simulink model "couple"  (R2024b)
settings: Solver=VariableStepAuto  StartTime=0.0  StopTime=10.0  RelTol=1e-3
undefined symbols (not defined in the file): rational, S, sparameters
libraries: simrfV2util1 x3, simrfV2elements x1, simrfV2junction1 x1, simrfV2sources1 x1

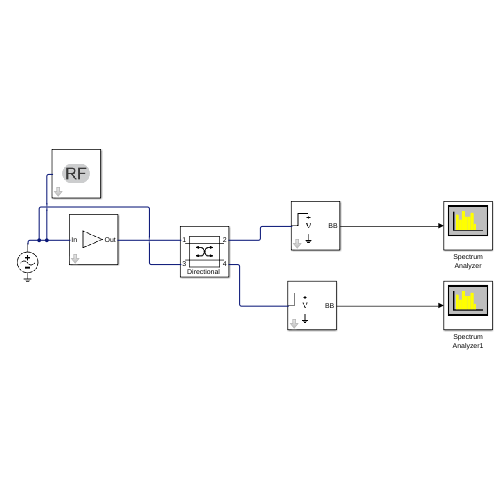
[thumbnail: Simulink's stored preview of the top-level diagram]
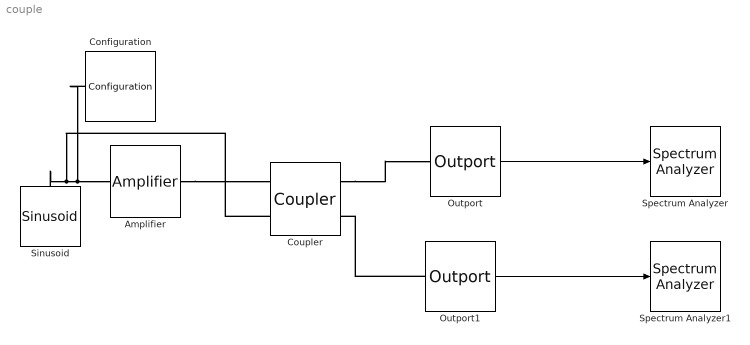
== system couple ==
  Amplifier : simrfV2elements/Amplifier  classname=amplifier  DataSource=Data file  File=unitygain.s2p  isNetworkObj=off  NetworkObject=sparameters('default.s2p')  Paramtype=S-parameters  Sparam=[0 0;1 0]  SparamFreq=1e9 Hz  SparamZ0=50  isRationalObj=off  RationalObject=rational('default.s2p')  Residues=0  Poles=0  DF={0 0; 1 0}  Source_linear_gain=Available power gain  linear_gain=100 dB  AmAmAmPmTable=[-25,5,-1;-10,20,-2;0,27,5;5,28,12]  Zin=50  Zout=50  Source_Poly=Even and odd order  Poly_Coeffs=[0 1]  IPType=Output  IP2=inf dBm  IP3=inf dBm  P1dB=inf dBm  Psat=inf dBm  Gcomp=inf dBm  InternalGrounding=on  SourceFreq=Extracted from data source  PlotFreq=[1e9:1e6:3e9] Hz  PlotType=X-Y plane  YParam1=S(1,1)  YFormat1=Magnitude (dB)  YParam2=None  YFormat2=Magnitude (dB)  YOption=Linear  XOption=Linear  SparamRepresentation=Time domain  FitTol=-40  FitOpt=Fit individually  MaxPoles=48  AutoImpulseLength=on  ImpulseLength=1e-10 s  MagModeling=off  AddNoise=on  NoiseType=Noise figure  NoiseDist=White  NF=0  MinNF=0  Gopt=0  RN=0  CarrierFreq=0 Hz  NoiseAutoImpulseLength=on  NoiseImpulseLength=1e-10 s  ConstS21NL=off  OpFreq=1 GHz  SetOpFreqAsMaxS21=off
  Configuration : simrfV2util1/Configuration  AutoFreq=on  Tones=[] Hz  Harmonics=[]  NormalizeCarrierPower=on  SolverType=Auto  UseCCode=on  StepSize=1e-6 s  AddNoise=on  defaultRNG=on  Seed=0  Temperature=290.0 K  SolverDelFlag=0  AbsTol=1e-6  RelTol=1e-3  MaxIter=10  ErrorEstimationType=2-norm over all variables  EnableInterpFilter=on  HiddenFIRfilterControllerParam=off  SmallSignalApprox=off  AllSimFreqs=on  SimFreqs=[] Hz  SimFreqsInternal=[]  SamplesPerFrame=1
  Coupler : simrfV2junction1/Coupler  classname=couplers  DataSource=Network-parameters  NumPorts=4  DeviceCirculator=Circulator clockwise  DeviceDivider=T power divider  DeviceCoupler=Directional coupler  Paramtype=S-parameters  Sparam=[0 0 1; 1 0 0; 0 1 0]  SparamFreq=1e9 Hz  SparamZ0=50  Phase12=0  Phase33=0  Alpha=0  NumberDividerOutports=2  Coupling=0  Directivity=inf  InsertionLoss=inf  ReturnLoss=inf  InternalGrounding=on  SparamRepresentation=Frequency domain  FitOpt=Share all poles  FitTol=-40  MaxPoles=48
  Outport : simrfV2util1/Outport  SensorType=Ideal voltage  OutputFormat=Complex Baseband  CarrierFreq=1 GHz  ZL=Inf  InternalGrounding=on  StepSize=1e-6 s  AutoStep=on  HalfPolyphaseLength=12
  Outport1 : simrfV2util1/Outport  SensorType=Ideal voltage  OutputFormat=Complex Baseband  CarrierFreq=1 GHz  ZL=Inf  InternalGrounding=on  StepSize=1e-6 s  AutoStep=on  HalfPolyphaseLength=12
  Sinusoid : simrfV2sources1/Sinusoid  SineSourceType=Ideal voltage  VO_I=0 V  IO_I=0 A  VO_Q=0 V  IO_Q=0 A  VA_I=5 V  IA_I=0 A  VA_Q=0 V  IA_Q=0 A  Fmod=10 MHz  TD=0 s  CarrierFreq=1 GHz  InternalGrounding=on
  Spectrum Analyzer : SpectrumAnalyzer  Tag=simrfV2util1/Spectrum Analyzer  WindowPosition=[222.000000,6.000000,537.000000,500.000000,]  Visible=on  ScopeFrameLocation=window  Method=Welch  AveragingMethod=Exponential  YLimits=[-175.33972416,-101.79755368]  AllowFFTLengthLessThanSamplesPerUpdate=on
  Spectrum Analyzer1 : SpectrumAnalyzer  Tag=simrfV2util1/Spectrum Analyzer  WindowPosition=[-90.000000,-426.000000,601.000000,500.000000,]  Visible=on  ScopeFrameLocation=window  Method=Welch  AveragingMethod=Exponential  YLimits=[-69.31912425,4.22304623]  AllowFFTLengthLessThanSamplesPerUpdate=on
  wires:
  Outport/1 -> Spectrum Analyzer/1
  Outport1/1 -> Spectrum Analyzer1/1
  connections:
  Sinusoid/LConn1 -- Coupler/LConn2 -- Configuration/LConn1 -- Amplifier/LConn1
  Amplifier/RConn1 -- Coupler/LConn1
  Coupler/RConn1 -- Outport/LConn1
  Outport1/LConn1 -- Coupler/RConn2
